simulink model "IMU_simulink_model"  (R2021a)
settings: Solver=VariableStepAuto  StartTime=0.0  StopTime=10.0  RelTol=1e-3
libraries: mspsensorlib x2, mspfiltlib x1, simulink_extras x1
settings Model: Creator=mynam  LastModifiedBy=mynam

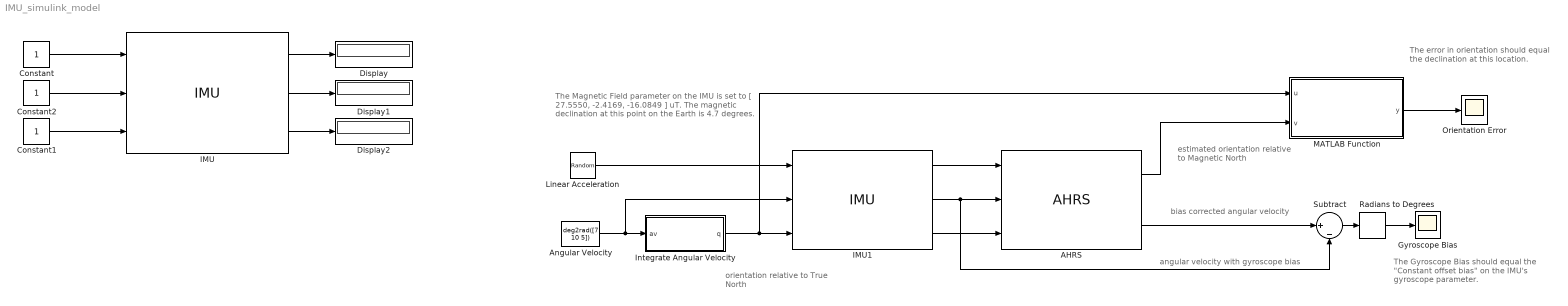
== system IMU_simulink_model ==
  note: estimated orientation
      | relative to Magnetic North
  note: The error in orientation should
      | equal the declination at this location.
  note: The Magnetic Field parameter on the IMU is set to
      | [ 27.5550, -2.4169, -16.0849 ] uT.
      |
      | The magnetic declination at this point
      | on the Earth is  4.7 degrees.
  note: bias corrected angular velocity
  note: angular velocity with gyroscope bias
  note: orientation relative
      | to True North
  note: The Gyroscope Bias should
      | equal the "Constant offset bias"
      | on the IMU's gyroscope parameter.
  AHRS : mspfiltlib/AHRS  DispRefFrame=NED  DecimationFactor=1  InitialProcessNoise=ahrsfilter.defaultProcessNoise  OrientationFormat=quaternion  SimulateUsing=Code generation  AccelerometerNoise=0.0001924722  GyroscopeNoise=9.1385e-5  MagnetometerNoise=0.1  GyroscopeDriftNoise=3.0462e-13  LinearAccelerationNoise=0.0096236100000000012  MagneticDisturbanceNoise=0.5  LinearAccelerationDecayFactor=0.5  MagneticDisturbanceDecayFactor=0.5  ExpectedMagneticFieldStrength=50
      settings: SourceProductBaseCode=TF,NV
  Angular Velocity : Constant  Value=deg2rad([7 10 5])  VectorParams1D=off  SampleTime=1/2
  Constant : Constant
  Constant1 : Constant
  Constant2 : Constant
  Display : Display
  Display1 : Display
  Display2 : Display
  Gyroscope Bias : Scope
  IMU : mspsensorlib/IMU  DispRefFrame=NED  Temperature=25  MagneticFieldNED=[ 27.5550, -2.4169, -16.0849 ]  MagneticFieldENU=[ -2.4169, 27.5550, 16.0849 ]  SeedDouble=67  SimulateUsing=Interpreted execution  AccelParamsMeasurementRange=Inf  AccelParamsResolution=0  AccelParamsConstantBias=[ 0, 0, 0 ]  AccelParamsAxesMisalignment=[ 0, 0, 0 ]  AccelParamsNoiseDensity=[ 0, 0, 0 ]  AccelParamsBiasInstability=[ 0, 0, 0 ]  AccelParamsRandomWalk=[ 0, 0, 0 ]  AccelParamsTemperatureBias=[ 0, 0, 0 ]  AccelParamsTemperatureScaleFactor=[ 0, 0, 0 ]  GyroParamsMeasurementRange=Inf  GyroParamsResolution=0  GyroParamsConstantBias=[ 0, 0, 0 ]  GyroParamsAxesMisalignment=[ 0, 0, 0 ]  GyroParamsAccelerationBias=[ 0, 0, 0 ]  GyroParamsNoiseDensity=[ 0, 0, 0 ]  GyroParamsBiasInstability=[ 0, 0, 0 ]  GyroParamsRandomWalk=[ 0, 0, 0 ]  GyroParamsTemperatureBias=[ 0, 0, 0 ]  GyroParamsTemperatureScaleFactor=[ 0, 0, 0 ]  MagParamsMeasurementRange=Inf  MagParamsResolution=0  MagParamsConstantBias=[ 0, 0, 0 ]  MagParamsAxesMisalignment=[ 0, 0, 0 ]  MagParamsNoiseDensity=[ 0, 0, 0 ]  MagParamsBiasInstability=[ 0, 0, 0 ]  MagParamsRandomWalk=[ 0, 0, 0 ]  MagParamsTemperatureBias=[ 0, 0, 0 ]  MagParamsTemperatureScaleFactor=[ 0, 0, 0 ]
      settings: SourceProductBaseCode=TF,NV
  IMU1 : mspsensorlib/IMU  DispRefFrame=NED  Temperature=25  MagneticFieldNED=[ 27.5550, -2.4169, -16.0849 ]  MagneticFieldENU=[ -2.4169, 27.5550, 16.0849 ]  SeedDouble=67  SimulateUsing=Code generation  AccelParamsMeasurementRange=19.613  AccelParamsResolution=0.0023928  AccelParamsConstantBias=[0.19 0.19 0.19]  AccelParamsAxesMisalignment=[0 0 0]  AccelParamsNoiseDensity=[0.0012356 0.0012356 0.0012356]  AccelParamsBiasInstability=[0 0 0]  AccelParamsRandomWalk=[0 0 0]  AccelParamsTemperatureBias=[0 0 0]  AccelParamsTemperatureScaleFactor=[0 0 0]  GyroParamsMeasurementRange=4.3633  GyroParamsResolution=0.0011  GyroParamsConstantBias=[0.0545 0.0545 0.0545]  GyroParamsAxesMisalignment=1.5  GyroParamsAccelerationBias=[0 0 0]  GyroParamsNoiseDensity=[0.00043633 0.00043633 0.00043633]  GyroParamsBiasInstability=[0 0 0]  GyroParamsRandomWalk=[0 0 0]  GyroParamsTemperatureBias=[0 0 0]  GyroParamsTemperatureScaleFactor=[0 0 0]  MagParamsMeasurementRange=1000  MagParamsResolution=0.1  MagParamsConstantBias=0  MagParamsAxesMisalignment=[0 0 0]  MagParamsNoiseDensity=[0.0424 0.0424 0.0424]  MagParamsBiasInstability=[0 0 0]  MagParamsRandomWalk=[0 0 0]  MagParamsTemperatureBias=[0 0 0]  MagParamsTemperatureScaleFactor=[0 0 0]
      settings: SourceProductBaseCode=TF,NV
  Integrate Angular Velocity : MATLAB Function  TreatAsAtomicUnit=on  mask{rate=2}
      mask prompts: rate "Sample Rate"
  Linear Acceleration : RandomNumber  Mean=[0 0 0]  SampleTime=1/2  VectorParams1D=off
  MATLAB Function : MATLAB Function  TreatAsAtomicUnit=on
  Orientation Error : Scope
  Radians to Degrees : simulink_extras/Transformations/Radians to Degrees
  Subtract : Sum  Inputs=||+|-
  wires:
  Constant/1 -> IMU/1
  Constant2/1 -> IMU/2
  Constant1/1 -> IMU/3
  IMU/1 -> Display/1
  IMU/2 -> Display1/1
  IMU/3 -> Display2/1
  AHRS/1 -> MATLAB Function/2(v)
  AHRS/2 -> Subtract/1
  IMU1/2 -> Subtract/2, AHRS/2
  MATLAB Function/1(y) -> Orientation Error/1
  Subtract/1 -> Radians to Degrees/1
  Angular Velocity/1 -> IMU1/2, Integrate Angular Velocity/1(av)
  Integrate Angular Velocity/1(q) -> MATLAB Function/1(u), IMU1/3
  Radians to Degrees/1 -> Gyroscope Bias/1
  Linear Acceleration/1 -> IMU1/1
  IMU1/1 -> AHRS/1
  IMU1/3 -> AHRS/3

== matlab function IMU_simulink_model/Integrate Angular Velocity ==
  data: av input; q output; rate parameter
function q = integrateAngVel(av, rate)
%INTEGRATEANGVEL Integrate angular velocity to a quaternion
%  Treat Angular Velocity as an incremental rotation vector.

%   Copyright 2019 The MathWorks, Inc.   

persistent orient
if isempty(orient)
    % Initial orientation is the identity quaternion.
    orient = cast(quaternion(1,0,0,0), 'like', av);
end

% Convert angular velocity to a rotation vector.
rv = quaternion(av*(1/rate), 'rotvec');
orient = rv * orient;
q = compact(orient);

== matlab function IMU_simulink_model/MATLAB Function ==
  data: u input; y output; v input
function y = orientationError(u,v)
%ORIENTATIONERROR Compute the quaternion distance in degrees

%   Copyright 2019 The MathWorks, Inc.   

y = rad2deg(dist(quaternion(u), quaternion(v)));
